simulink model "uwb_3_nature16"  (R2025a)
settings: Solver=VariableStepAuto  StartTime=0.0  StopTime=1e-7  RelTol=1e-3
undefined symbols (not defined in the file or in its folder): dspblkCoreblockFVToolHelper, gcbh
libraries: commdigbbndpm3 x4, dspfiltersrcs x2, dspfdesign x2, dspstat3 x2, simulink x2, commrfcorlib x1, dspsigops x1
settings Model: Creator=IWMAI  LastModifiedBy=IWMAI

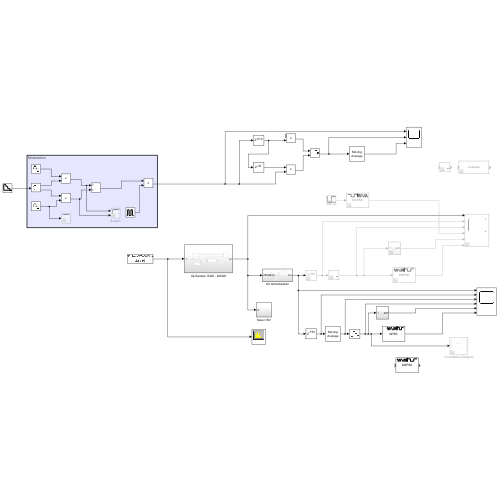
[thumbnail: Simulink's stored preview of the top-level diagram]
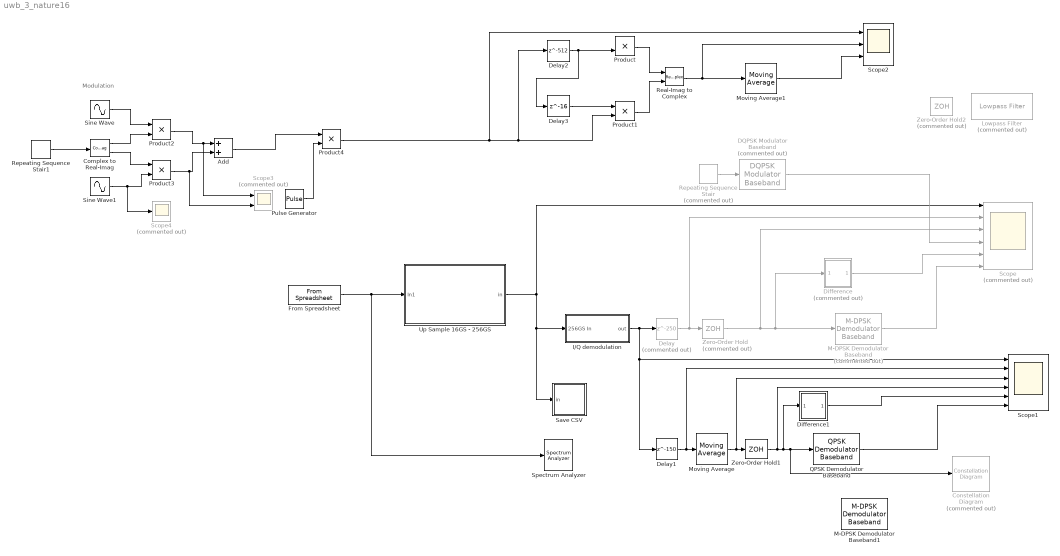
== system uwb_3_nature16 ==
  note: Modulation
  Add : Sum
  Complex to Real-Imag : ComplexToRealImag
  Constellation Diagram : ConstellationDiagram  Commented=on  WindowPosition=[724.000000,276.000000,600.000000,600.000000,]  ScopeFrameLocation=window  SymbolsToDisplaySource=Property  SymbolsToDisplay=2500  DefaultConfigurationName=comm.scopes.ConstellationDiagramBlockCfg
  DQPSK Modulator Baseband : commdigbbndpm3/DQPSK Modulator Baseband  Commented=on  InType=Integer  Enc=Gray  Ph=0  outDtype=double
  Delay : Delay  Commented=on  DelayLength=250
  Delay1 : Delay  DelayLength=150
  Delay2 : Delay  DelayLength=512
  Delay3 : Delay  DelayLength=16
  Difference : Subsystem  Commented=on
  Difference1 : Subsystem
  From Spreadsheet : FromSpreadsheet  FileName=C:\Users\IWMAI\University of Toronto\Yu Huang - Summer-2025-sharted\Yongkang\v3_250617\csv\data16.csv  SheetName=data16  OutDataTypeStr=double  SampleTime=1/16e9
  I/Q demodulation : Subsystem
  Lowpass Filter : dspfdesign/Lowpass Filter  Commented=on  FilterType=FIR  DesignForMinimumOrder=on  FilterOrder=50  PassbandFrequency=1/128  StopbandFrequency=1/64  PassbandRipple=0.1  StopbandAttenuation=80  SampleRateMode=Use normalized frequency (0 to 1)  SampleRate=44100  SimulateUsing=Interpreted execution  roundingMode=Floor  coeffsDataTypeStr=fixdt(1,16)
  M-DPSK Demodulator Baseband : commdigbbndpm3/M-DPSK Demodulator Baseband  Commented=on  M=4  OutType=Integer  Dec=Gray  Ph=0  outDtype1=Inherit via internal rule  outDtype2=Inherit via internal rule
  M-DPSK Demodulator Baseband1 : commdigbbndpm3/M-DPSK Demodulator Baseband  M=4  OutType=Integer  Dec=Gray  Ph=0  outDtype1=Inherit via internal rule  outDtype2=Inherit via internal rule
  Moving Average : dspstat3/Moving Average  Method=Sliding window  ForgettingFactorPort=off  SpecifyWindowLength=on  WindowLength=100  OverlapLength=99  AllowArbitraryInputLength=off  ForgettingFactor=0.9  SimulateUsing=Interpreted execution
  Moving Average1 : dspstat3/Moving Average  Method=Sliding window  ForgettingFactorPort=off  SpecifyWindowLength=on  WindowLength=256  OverlapLength=255  AllowArbitraryInputLength=off  ForgettingFactor=0.9  SimulateUsing=Interpreted execution
  Product{,1..4} (5 alike) : Product
  Pulse Generator : DiscretePulseGenerator  PulseType=Time based  Period=1/500e6  PulseWidth=37.5  PhaseDelay=1/256e9  SampleTime=0.000001
  QPSK Demodulator Baseband : commdigbbndpm3/QPSK Demodulator Baseband  OutType=Integer  DecType=Hard decision  VarSource=Dialog  Variance=1  Dec=Binary  Ph=pi/4  outDtype1=Inherit via internal rule  outDtype2=Inherit via internal rule  derotateFactorWordLen=16  derotateFactorDataTypeStr=Inherit: Same word length as input  derotateFactorLastDataTypeStr=Inherit: Same word length as input
      settings: LibrarySourceBlock=|
      | commhdldigbbndpm/QPSK
      | Demodulator
      | Baseband
  Real-Imag to Complex : RealImagToComplex
  Repeating Sequence Stair : simulink/Sources/Repeating Sequence Stair  Commented=on  OutValues=[0 2].'  tsamp=1/500003519.873597  OutMin=[]  OutMax=[]  OutDataTypeStr=double  OutputDataTypeScalingMode=double  OutDataType=fixdt(0,8)  ConRadixGroup=Best Precision: Vector-wise  OutScaling=2^-12
  Repeating Sequence Stair1 : simulink/Sources/Repeating Sequence Stair  OutValues=[3 3 2 2 1 1 0 0].'  tsamp=1/500003519.873597  OutMin=[]  OutMax=[]  OutDataTypeStr=double  OutputDataTypeScalingMode=double  OutDataType=fixdt(0,8)  ConRadixGroup=Best Precision: Vector-wise  OutScaling=2^-12
  Save CSV : Subsystem
  Scope : Scope  Commented=on  NumInputPorts=6
      settings: ActiveDisplayYMinimum=-4.6231372013846705  ActiveDisplayYMaximum=4.7306324654418139
  Scope1 : Scope  NumInputPorts=6
      settings: ActiveDisplayYMinimum=-1.8698047125750872  ActiveDisplayYMaximum=3.6095755689182307  DataLoggingVariableName=ScopeData3
  Scope2 : Scope  NumInputPorts=3
      settings: ActiveDisplayYMinimum=-7.8536631620890986  ActiveDisplayYMaximum=6.9997378876221186  DataLoggingVariableName=ScopeData2
  Scope3 : Scope  Commented=on  NumInputPorts=2
      settings: ActiveDisplayYMinimum=-1  ActiveDisplayYMaximum=1  DataLoggingVariableName=ScopeData5
  Scope4 : Scope  Commented=on
      settings: ActiveDisplayYMinimum=-6.9684119114826721  ActiveDisplayYMaximum=6.352909516611934  DataLoggingVariableName=ScopeData4
  Sine Wave : Sin  Frequency=2*pi*4e9  Phase=pi/2  SampleTime=1/256e9
  Sine Wave1 : Sin  Frequency=2*pi*4e9  SampleTime=1/256e9
  Spectrum Analyzer : SpectrumAnalyzer  WindowPosition=[251.000000,-1103.000000,1536.000000,793.000000,]  ScopeFrameLocation=window  WindowInvariantSamplesPerUpdate=on  Span=15999999999.999998  StartFrequency=-7999999999.999999  StopFrequency=7999999999.999999  YLimits=[-138.8302 11.7855]  SelectedToolstripTab=spectrumAnalyzerToolstrip.channelMeasurementsTab
      settings: OpenAtSimulationStart=off
  Up Sample 16GS - 256GS : Subsystem
  Zero-Order Hold : ZeroOrderHold  Commented=on  SampleTime=1/500003519.873597
  Zero-Order Hold1 : ZeroOrderHold  SampleTime=1/500003519.873597
  Zero-Order Hold2 : ZeroOrderHold  Commented=on  SampleTime=-1
  wires:
  From Spreadsheet/1 -> Spectrum Analyzer/1, Up Sample 16GS - 256GS/1(In1)
  I/Q demodulation/1(out) -> Scope1/1, Delay1/1, Delay/1
  Zero-Order Hold/1 -> Scope/3, M-DPSK Demodulator Baseband/1, Difference/1(In1)
  Repeating Sequence Stair/1 -> DQPSK Modulator Baseband/1
  Difference/1(diff) -> Scope/5
  Up Sample 16GS - 256GS/1(in) -> Scope/1, Save CSV/1(in), I/Q demodulation/1(256GS In)
  M-DPSK Demodulator Baseband/1 -> Scope/6
  DQPSK Modulator Baseband/1 -> Scope/4
  Delay/1 -> Scope/2, Zero-Order Hold/1
  Delay1/1 -> Scope1/2, Moving Average/1
  Moving Average/1 -> Scope1/3, Zero-Order Hold1/1
  Zero-Order Hold1/1 -> Scope1/4, Constellation Diagram/1, QPSK Demodulator Baseband/1, Difference1/1(In1)
  Difference1/1(diff) -> Scope1/5
  QPSK Demodulator Baseband/1 -> Scope1/6
  Delay2/1 -> Delay3/1, Product/2
  Delay3/1 -> Product1/1
  Product/1 -> Real-Imag to Complex/1
  Product1/1 -> Real-Imag to Complex/2
  Real-Imag to Complex/1 -> Moving Average1/1, Scope2/2
  Moving Average1/1 -> Scope2/3
  Pulse Generator/1 -> Product4/2
  Complex to Real-Imag/2 -> Product3/1
  Product3/1 -> Scope3/2, Add/2
  Sine Wave1/1 -> Scope4/1, Product3/2
  Add/1 -> Product4/1
  Complex to Real-Imag/1 -> Product2/2
  Product2/1 -> Scope3/1, Add/1
  Sine Wave/1 -> Product2/1
  Repeating Sequence Stair1/1 -> Complex to Real-Imag/1
  Product4/1 -> Scope2/1, Delay2/1, Product1/2

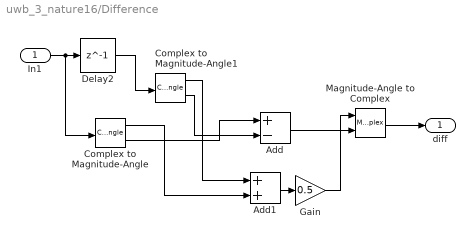
== system uwb_3_nature16/Difference ==
  In1 : Inport
  Add : Sum  Inputs=+-
  Add1 : Sum
  Complex to Magnitude-Angle : ComplexToMagnitudeAngle
  Complex to Magnitude-Angle1 : ComplexToMagnitudeAngle
  Delay2 : Delay  DelayLength=1
  Gain : Gain  Gain=0.5
  Magnitude-Angle to Complex : MagnitudeAngleToComplex
  diff : Outport
  wires:
  Gain/1 -> Magnitude-Angle to Complex/1
  Complex to Magnitude-Angle1/2 -> Add/2
  Add1/1 -> Gain/1
  Add/1 -> Magnitude-Angle to Complex/2
  Complex to Magnitude-Angle/2 -> Add/1
  Magnitude-Angle to Complex/1 -> diff/1
  Complex to Magnitude-Angle/1 -> Add1/2
  Complex to Magnitude-Angle1/1 -> Add1/1
  Delay2/1 -> Complex to Magnitude-Angle1/1
  In1/1 -> Delay2/1, Complex to Magnitude-Angle/1

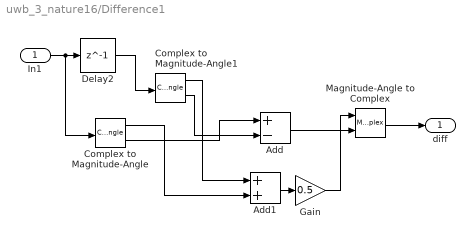
== system uwb_3_nature16/Difference1 ==
  In1 : Inport
  Add : Sum  Inputs=+-
  Add1 : Sum
  Complex to Magnitude-Angle : ComplexToMagnitudeAngle
  Complex to Magnitude-Angle1 : ComplexToMagnitudeAngle
  Delay2 : Delay  DelayLength=1
  Gain : Gain  Gain=0.5
  Magnitude-Angle to Complex : MagnitudeAngleToComplex
  diff : Outport
  wires:
  Gain/1 -> Magnitude-Angle to Complex/1
  Complex to Magnitude-Angle1/2 -> Add/2
  Add1/1 -> Gain/1
  Add/1 -> Magnitude-Angle to Complex/2
  Complex to Magnitude-Angle/2 -> Add/1
  Magnitude-Angle to Complex/1 -> diff/1
  Complex to Magnitude-Angle/1 -> Add1/2
  Complex to Magnitude-Angle1/1 -> Add1/1
  Delay2/1 -> Complex to Magnitude-Angle1/1
  In1/1 -> Delay2/1, Complex to Magnitude-Angle/1

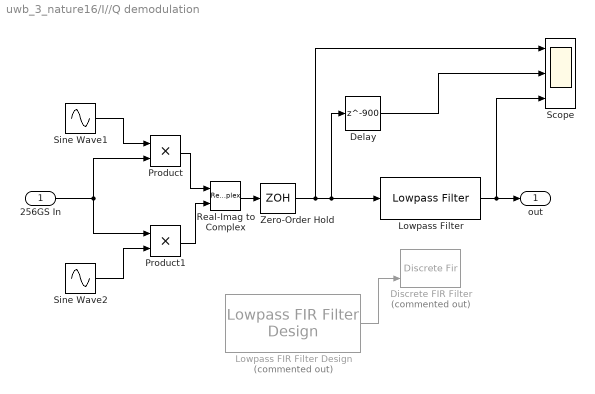
== system uwb_3_nature16/I//Q demodulation ==
  256GS In : Inport
  Delay : Delay  DelayLength=900
  Discrete FIR Filter : DiscreteFir  Commented=on  LoadFcn=dspblkCoreblockFVToolHelper(gcbh,'load');  CoefSource=Input port
      settings: CopyFcn=dspblkCoreblockFVToolHelper(gcbh,'copy');  DeleteFcn=dspblkCoreblockFVToolHelper(gcbh,'close');  ModelCloseFcn=dspblkCoreblockFVToolHelper(gcbh,'close');  PreSaveFcn=dspblkCoreblockFVToolHelper(gcbh,'presave');  PostSaveFcn=dspblkCoreblockFVToolHelper(gcbh,'postsave');  CloseFcn=dspblkCoreblockFVToolHelper(gcbh,'close');  InputPortMap=u0,u1
  Lowpass FIR Filter Design : dspfiltersrcs/Lowpass FIR Filter Design  Commented=on  SmoothParameters=off  SmoothingFactor=0.6  FilterOrderPort=off  FilterOrder=100  MaxOrder=100  CutoffFrequencyPort=off  CutoffFrequency=1/256e9  Window=Hann  SidelobeAttenuationPort=off  SidelobeAttenuation=60  KaiserWindowParameterPort=off  KaiserWindowParameter=.5  OutputDataType=double  SampleTime=1/256e9  SimulateUsing=Interpreted execution
      settings: LibrarySourceBlock=dspfdesign/Lowpass FIR Filter Design
  Lowpass Filter : dspfdesign/Lowpass Filter  FilterType=FIR  DesignForMinimumOrder=on  FilterOrder=50  PassbandFrequency=1/64  StopbandFrequency=1/32  PassbandRipple=0.1  StopbandAttenuation=80  SampleRateMode=Use normalized frequency (0 to 1)  SampleRate=44100  SimulateUsing=Interpreted execution  roundingMode=Floor  coeffsDataTypeStr=fixdt(1,16)
  Product : Product
  Product1 : Product
  Real-Imag to Complex : RealImagToComplex
  Scope : Scope  NumInputPorts=3
      settings: ActiveDisplayYMinimum=-3.8072894106917321  ActiveDisplayYMaximum=4.4801769671043541  DataLoggingVariableName=ScopeData2
  Sine Wave1 : Sin  Frequency=2 * pi * 4e9  Phase=pi/2  SampleTime=0
  Sine Wave2 : Sin  Frequency=2 * pi * 4e9  SampleTime=0
  Zero-Order Hold : ZeroOrderHold  SampleTime=1/256e9
  out : Outport
  wires:
  256GS In/1 -> Product/2, Product1/1
  Sine Wave2/1 -> Product1/2
  Sine Wave1/1 -> Product/1
  Product/1 -> Real-Imag to Complex/1
  Product1/1 -> Real-Imag to Complex/2
  Lowpass FIR Filter Design/1 -> Discrete FIR Filter/2
  Lowpass Filter/1 -> Scope/3, out/1
  Real-Imag to Complex/1 -> Zero-Order Hold/1
  Zero-Order Hold/1 -> Scope/1, Delay/1, Lowpass Filter/1
  Delay/1 -> Scope/2

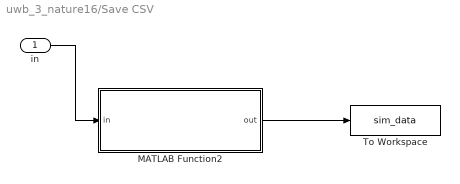
== system uwb_3_nature16/Save CSV ==
  in : Inport
  MATLAB Function2 : MATLAB Function  TreatAsAtomicUnit=on
  To Workspace : ToWorkspace  VariableName=sim_data  SaveFormat=Timeseries  SampleTime=-1
  wires:
  MATLAB Function2/1(out) -> To Workspace/1
  in/1 -> MATLAB Function2/1(in)

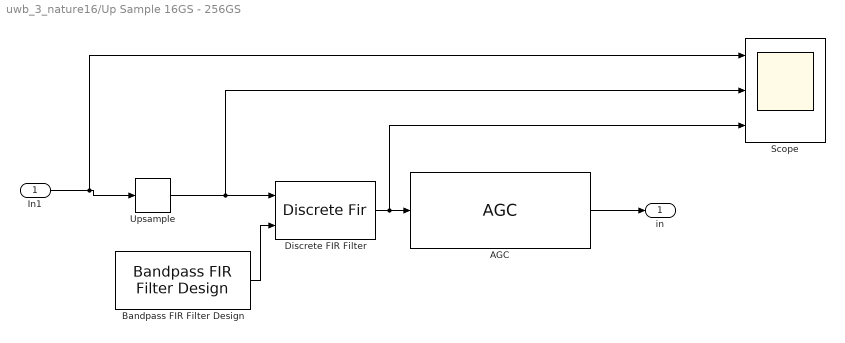
== system uwb_3_nature16/Up Sample 16GS - 256GS ==
  In1 : Inport
  AGC : commrfcorlib/AGC  LegacyMode=off  DetectorMethod=Rectifier  LoopMethod=Linear  UpdatePeriod=100  StepSize=0.1  AdaptationStepSize=0.01  DesiredOutputPower=1  AveragingLength=512  MaximumGain=30  MaxPowerGain=60  GainOutputPort=off  InputPowerOutputPort=off  SimulateUsing=Interpreted execution
  Bandpass FIR Filter Design : dspfiltersrcs/Bandpass FIR Filter Design  SmoothParameters=off  SmoothingFactor=0.6  FilterOrderPort=off  FilterOrder=100  MaxOrder=100  CenterFrequencyPort=off  CenterFrequency=1/64  BandwidthPort=off  Bandwidth=0.01  Window=Hann  SidelobeAttenuationPort=off  SidelobeAttenuation=60  KaiserWindowParameterPort=off  KaiserWindowParameter=.5  OutputDataType=double  SampleTime=256e9  SimulateUsing=Interpreted execution
      settings: LibrarySourceBlock=dspfdesign/Bandpass FIR Filter Design
  Discrete FIR Filter : DiscreteFir  LoadFcn=dspblkCoreblockFVToolHelper(gcbh,'load');  CoefSource=Input port
      settings: CopyFcn=dspblkCoreblockFVToolHelper(gcbh,'copy');  DeleteFcn=dspblkCoreblockFVToolHelper(gcbh,'close');  ModelCloseFcn=dspblkCoreblockFVToolHelper(gcbh,'close');  PreSaveFcn=dspblkCoreblockFVToolHelper(gcbh,'presave');  PostSaveFcn=dspblkCoreblockFVToolHelper(gcbh,'postsave');  CloseFcn=dspblkCoreblockFVToolHelper(gcbh,'close');  InputPortMap=u0,u1
  Scope : Scope  NumInputPorts=3
      settings: ActiveDisplayYMinimum=-0.1766463393208148  ActiveDisplayYMaximum=0.16150855826432609
  Upsample : dspsigops/Upsample  FactorSource=Dialog parameter  N=16  Nmax=16  phase=0  RateOptions=Allow multirate processing  ic=0  mode=Unused parameter value
      settings: LibrarySourceBlock=dsphdlsupportsigops/Upsample
  in : Outport
  wires:
  Upsample/1 -> Scope/2, Discrete FIR Filter/1
  Discrete FIR Filter/1 -> Scope/3, AGC/1
  AGC/1 -> in/1
  Bandpass FIR Filter Design/1 -> Discrete FIR Filter/2
  In1/1 -> Scope/1, Upsample/1

== matlab function uwb_3_nature16/Save CSV/MATLAB Function2 ==
  data: in input; out output
function out = save_csv(in)
%#codegen
% This function processes one sample at a time.
% To store data across simulation steps, you need to use persistent variables.

persistent data_buffer;
persistent index_counter;

if isempty(data_buffer)
    % Initialize buffer and counter when simulation starts or resets
    data_buffer = zeros(0, 2); % Column 1 for index, Column 2 for data
    index_counter = 0;
end

% Increment index and store current sample
index_counter = index_counter + 1;
data_buffer = [data_buffer; index_counter, in];

% Output the current sample (or anything else you need downstream)
out = in;

% You can add logic here to write to CSV periodically,
% but it's generally better to do it after simulation.
% For this method, we'll let 'To Workspace' handle saving.

% At the end of simulation, the persistent variables will be cleared unless
% you explicitly save them or access them from the base workspace.
% For 'To Workspace' method, it's about the *output* of this block.
end
